simulink model "template_rotary_inverted_pendulum_2021b"  (R2021b)
settings: Solver=FixedStepDiscrete  StartTime=0.0  StopTime=inf  FixedStep=0.005  RelTol=1e-3
undefined symbols (not defined in the file or in its folder): K, National_Instruments, PCI
libraries: simulink_extras x3, sldrtlib x2
settings Model: SimulationMode=external  ExtModeTrigDuration=200000  Creator=magudelo  LastModifiedBy=viking
settings SolverCC: AlgebraicLoopSolver=TrustRegion  InsertRTBMode=Always
settings DataIOCC: LimitDataPoints=on  SaveFormat=Array  SignalLoggingSaveFormat=ModelDataLogs  ReturnWorkspaceOutputs=off
settings OptimizationCC: ExpressionDepthLimit=2147483647
settings DebuggingCC: UnderspecifiedInitializationDetection=Classic  MergeDetectMultiDrivingBlocksExec=none  SolverPrmCheckMsg=warning  FcnCallInpInsideContextMsg=warning  StateNameClashWarn=warning  PregeneratedLibrarySubsystemCodeDiagnostic=none  SFUnexpectedBacktrackingDiag=warning  SFNoUnconditionalDefaultTransitionDiag=warning  SFExecutionAtInitializationDiag=none  SFMachineParentedDataDiag=warning  ArithmeticOperatorsInVariantConditions=warning
settings ModelReferenceCC: PropagateSignalLabelsOutOfModel=off
settings SFSimCC: SimUseLocalCustomCode=off  CustomCodeUndefinedFunction=UseInterfaceOnly
settings RTWCC: Description=Simulink Desktop Real-Time  SystemTargetFile=sldrt.tlc  TemplateMakefile=sldrt.tmf  RTWUseLocalCustomCode=off  RTWCompilerOptimization=on
settings CodeAppCC: MaxIdLength=95  StateflowObjectComments=on
settings SimulinkDesktopRealTimeCC: TargetPreCompLibLocation=C:\Program Files\MATLAB\R2021b\toolbox\sldrt\lib\win64  TargetLangStandard=C89/C90 (ANSI)  SupportVariableSizeSignals=off
settings ConfigComp: CovMetricSettings=dw  CovSaveCumulativeToWorkspaceVar=on  CovSaveSingleToWorkspaceVar=on  CovExternalEMLEnable=off

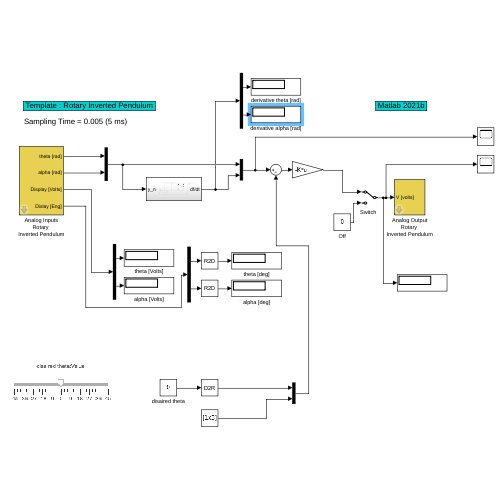
[thumbnail: Simulink's stored preview of the top-level diagram]
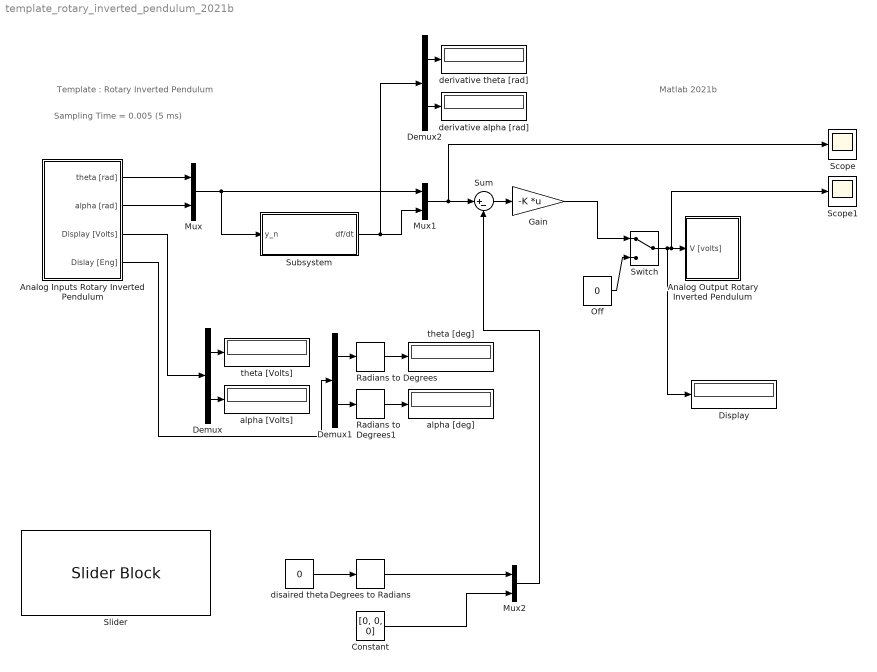
== system template_rotary_inverted_pendulum_2021b ==
  note: Matlab 2021b
  note: Sampling Time = 0.005 (5 ms)
  note: Template : Rotary Inverted Pendulum
  Analog Inputs Rotary Inverted Pendulum : Subsystem  mask(Analog Inputs. Rotary Inverted Pendulum){factor_theta=0.5959, offset_theta=-1.7, factor_alfa=0.3, offset_alfa=0.67}
      mask prompts: factor_theta "F_theta = Convertion factor from Volts to Radians (theta) :"; offset_theta "Off_theta = Offset for the angle of the arm (Volts):"; factor_alfa "F_alpha = Convertion Factor From Volts to Radians (alfa) :"; offset_alfa "Off_alpha = Offset for the angle of the rob (Volts) :"
      mask help:
      | Remember:
      |    Angle of the arm (theta) => channel ACH0
      |    Angle of the rod (alpha)    => channel ACH1
      |
      |   Angle of the arm  [rad] = F_theta * ( Angle of the arm [v]  + off_theta )
      |   Angle of the rod [rad] = F_alpha * ( Angle of the rod [v] + off_alpha )
  Analog Output Rotary Inverted Pendulum : Subsystem  mask(Analog Output - Rotary Inverted Pendulum){}
      mask help:
      | Remember
      |    AO 0 => Power Amplifier + Motor
  Constant : Constant  Value=[0, 0, 0]
  Degrees to Radians : simulink_extras/Transformations/Degrees to Radians
  Demux : Demux  Outputs=2
  Demux1 : Demux  Outputs=2
  Demux2 : Demux  Outputs=2
  Display : Display
  Gain : Gain  Gain=-K  Multiplication=Matrix(K*u)
  Mux : Mux  Inputs=2
  Mux1 : Mux  Inputs=2
  Mux2 : Mux  Inputs=2
  Off : Constant  Value=0
  Radians to Degrees : simulink_extras/Transformations/Radians to Degrees
  Radians to Degrees1 : simulink_extras/Transformations/Radians to Degrees
  Scope : Scope
  Scope1 : Scope
  Slider : SliderBlock  ScaleMin=-45  ScaleMax=45
  Subsystem : Subsystem
  Sum : Sum  Inputs=|+-
  "Switch  " : ManualSwitch
  alpha [Volts] : Display
      settings: SampleTime=0.25
  alpha [deg] : Display
      settings: SampleTime=0.25
  derivative alpha [rad] : Display
      settings: SampleTime=0.25
  derivative theta [rad] : Display
      settings: SampleTime=0.25
  disaired theta : Constant  Value=0
  theta [Volts] : Display
      settings: SampleTime=0.25
  theta [deg] : Display
      settings: SampleTime=0.25
  wires:
  Demux/1 -> theta [Volts]/1
  Demux/2 -> alpha [Volts]/1
  Analog Inputs Rotary Inverted Pendulum/3(Display [Volts]) -> Demux/1
  Analog Inputs Rotary Inverted Pendulum/4(Dislay [Eng]) -> Demux1/1
  Off/1 -> "Switch  "/2
  "Switch  "/1 -> Display/1, Scope1/1, Analog Output Rotary Inverted Pendulum/1(V [volts])
  Demux1/1 -> Radians to Degrees/1
  Radians to Degrees/1 -> theta [deg]/1
  Demux1/2 -> Radians to Degrees1/1
  Radians to Degrees1/1 -> alpha [deg]/1
  Analog Inputs Rotary Inverted Pendulum/1(theta [rad]) -> Mux/1
  Analog Inputs Rotary Inverted Pendulum/2(alpha [rad]) -> Mux/2
  Mux/1 -> Subsystem/1(y_n), Mux1/1
  Gain/1 -> "Switch  "/1
  Mux1/1 -> Scope/1, Sum/1
  Sum/1 -> Gain/1
  Mux2/1 -> Sum/2
  Constant/1 -> Mux2/2
  Degrees to Radians/1 -> Mux2/1
  disaired theta/1 -> Degrees to Radians/1
  Subsystem/1(df/dt) -> Demux2/1, Mux1/2
  Demux2/1 -> derivative theta [rad]/1
  Demux2/2 -> derivative alpha [rad]/1

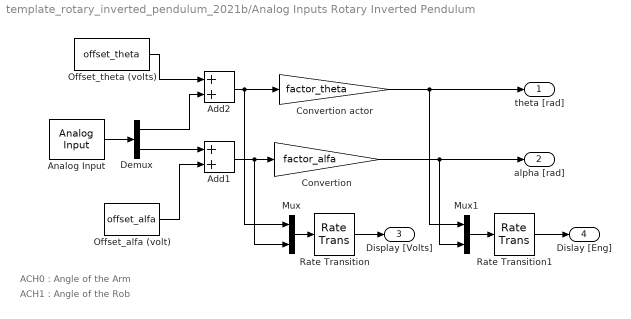
== system template_rotary_inverted_pendulum_2021b/Analog Inputs Rotary Inverted Pendulum ==
  note: ACH1 : Angle of the Rob
  note: ACH0 : Angle of the Arm
  Add1 : Sum
  Add2 : Sum
  Analog Input : sldrtlib/Analog Input  SampleTime=0.005  MaxMissedTicks=10  ShowMissedTicks=off  YieldWhenWaiting=off  DrvName=National_Instruments/PCI-6014  DrvAddress=4294967295  DrvOptions=[1 0 0 0 0 0]  Channels=[1 2]  RangeMode=1  VoltRange=1  DataType=1
      settings: AttributesFormatString=National Instruments\nPCI-6014 [auto]
  "Convertion " : Gain  Gain=factor_alfa
  Convertion actor : Gain  Gain=factor_theta
  Demux : Demux  Outputs=2
  Mux : Mux  Inputs=2
  Mux1 : Mux  Inputs=2
  Offset_alfa (volt) : Constant  Value=offset_alfa
  Offset_theta (volts) : Constant  Value=offset_theta
  Rate Transition : RateTransition  OutPortSampleTime=0.25
  Rate Transition1 : RateTransition  OutPortSampleTime=0.25
  theta [rad] : Outport  VectorParamsAs1DForOutWhenUnconnected=off
  alpha [rad] : Outport  Port=2  VectorParamsAs1DForOutWhenUnconnected=off
  Display [Volts] : Outport  Port=3  VectorParamsAs1DForOutWhenUnconnected=off
  Dislay [Eng] : Outport  Port=4  VectorParamsAs1DForOutWhenUnconnected=off
  wires:
  Rate Transition1/1 -> Dislay [Eng]/1
  Mux1/1 -> Rate Transition1/1
  Rate Transition/1 -> Display [Volts]/1
  Mux/1 -> Rate Transition/1
  "Convertion "/1 -> Mux1/2, alpha [rad]/1
  Add1/1 -> Mux/2, "Convertion "/1
  Offset_alfa (volt)/1 -> Add1/2
  Demux/2 -> Add1/1
  Convertion actor/1 -> Mux1/1, theta [rad]/1
  Offset_theta (volts)/1 -> Add2/1
  Add2/1 -> Mux/1, Convertion actor/1
  Demux/1 -> Add2/2
  Analog Input/1 -> Demux/1

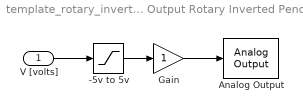
== system template_rotary_inverted_pendulum_2021b/Analog Output Rotary Inverted Pendulum ==
  V [volts] : Inport
  -5v to 5v : Saturate  UpperLimit=5  LowerLimit=-5
  Analog Output : sldrtlib/Analog Output  SampleTime=0.005  MaxMissedTicks=10  ShowMissedTicks=off  YieldWhenWaiting=off  DrvName=National_Instruments/PCI-6014  DrvAddress=4294967295  DrvOptions=[1 0 0 0 0 0]  Channels=1  RangeMode=1  VoltRange=1  InitialValue=0  FinalValue=0
      settings: AttributesFormatString=National Instruments\nPCI-6014 [auto]
  Gain : Gain
  wires:
  V [volts]/1 -> -5v to 5v/1
  -5v to 5v/1 -> Gain/1
  Gain/1 -> Analog Output/1

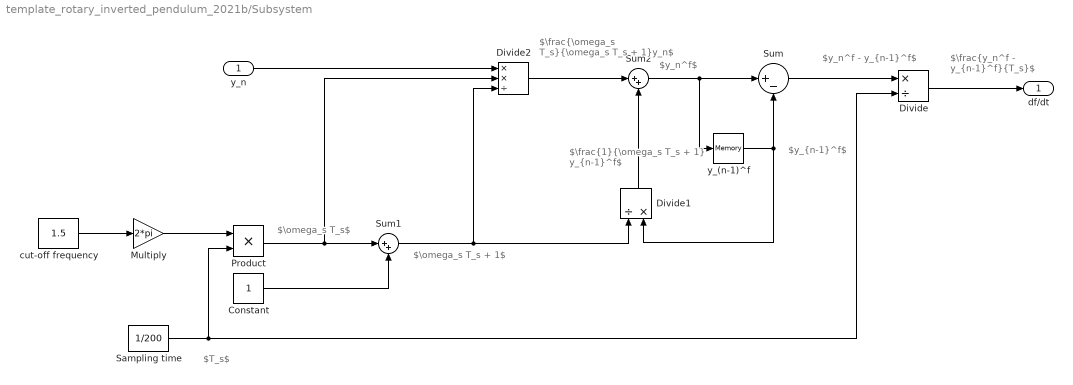
== system template_rotary_inverted_pendulum_2021b/Subsystem ==
  note: $y_n^f$
  note: $\frac{\omega_s T_s}{\omega_s T_s + 1}y_n$
  note: $y_n^f - y_{n-1}^f$
  note: $\omega_s T_s$
  note: $y_{n-1}^f$
  note: $\frac{1}{\omega_s T_s + 1} y_{n-1}^f$
  note: $\omega_s T_s + 1$
  note: $\frac{y_n^f - y_{n-1}^f}{T_s}$
  note: $T_s$
  y_n : Inport
  Constant : Constant
  Divide : Product  Inputs=*/
  Divide1 : Product  Inputs=/*
  Divide2 : Product  Inputs=**/
  Multiply : Gain  Gain=2*pi
  Product : Product
  Sampling time : Constant  Value=1/200
  Sum : Sum  Inputs=|+-
  Sum1 : Sum  Inputs=|++
  Sum2 : Sum  Inputs=|++
  cut-off frequency : Constant  Value=1.5
  y_(n-1)^f : Memory
  df/dt : Outport
  wires:
  Sum2/1 -> y_(n-1)^f/1, Sum/1
  Divide2/1 -> Sum2/1
  Sum1/1 -> Divide2/3, Divide1/1
  Divide/1 -> df/dt/1
  Sum/1 -> Divide/1
  y_(n-1)^f/1 -> Divide1/2, Sum/2
  Divide1/1 -> Sum2/2
  Product/1 -> Divide2/2, Sum1/1
  Sampling time/1 -> Product/2, Divide/2
  y_n/1 -> Divide2/1
  Constant/1 -> Sum1/2
  Multiply/1 -> Product/1
  cut-off frequency/1 -> Multiply/1
